simulink model "Cruise_Control_Reference"  (R2020b)
settings: Solver=VariableStepAuto  StartTime=0.0  StopTime=10.0  RelTol=1e-3
values from neighbouring files (symbols this model uses):
  b = 50.0    [Cruise_DataDictionary.sldd]
  m = 1000.0    [Cruise_DataDictionary.sldd]
settings Model: DataDictionary=Cruise_DataDictionary.sldd  Creator=Sourav Kumar  LastModifiedBy=Sourav Kumar
settings DataIOCC: SaveOutput=off  SaveTime=off

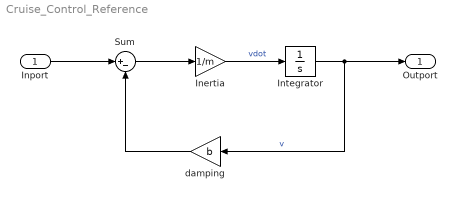
== system Cruise_Control_Reference ==
  Inport : Inport  OutDataTypeStr=double  PortDimensions=1  SampleTime=0
  Inertia : Gain  Gain=1/m
  Integrator : Integrator
  Sum : Sum  Inputs=|+-
  damping : Gain  Gain=b
  Outport : Outport  OutDataTypeStr=double  PortDimensions=1  SampleTime=0
  wires:
  Inport/1 -> Sum/1
  Inertia/1 -> Integrator/1  "vdot"
  Sum/1 -> Inertia/1
  Integrator/1 -> damping/1, Outport/1  "v"
  damping/1 -> Sum/2
